simulink model "debugController"  (R2017a)
settings: Solver=VariableStepAuto  StartTime=0.0  StopTime=10.0  RelTol=1e-3
values from neighbouring files (symbols this model uses):
  k_bal = 10    [automatas_matlab.m]
  m_c = 50000    [automatas_matlab.m]
  m_l = 65000    [automatas_matlab.m]
  M_t = m_c + (J_w_t + J_m_t * r_t ^ 2)/ R_w_t ^ 2    (= 59008)    [automatas_matlab.m]
  n_bal = 3    [automatas_matlab.m]
undefined symbols (not defined in the file or in its folder): Ba_b, Ksa_b, lh
settings Model: Creator=laure  LastModifiedBy=laure

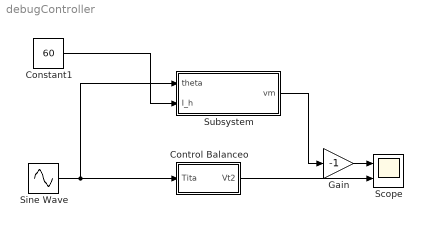
== system debugController ==
  Constant1 : Constant  Value=60
  Control Balanceo : Subsystem
  Gain : Gain  Gain=-1
  Scope : Scope  NumInputPorts=2
  Sine Wave : Sin  SampleTime=0
  Subsystem : Subsystem
  wires:
  Control Balanceo/1(Vt2) -> Scope/2
  Constant1/1 -> Subsystem/2(I_h)
  Sine Wave/1 -> Subsystem/1(theta), Control Balanceo/1(Tita)
  Subsystem/1(vm) -> Gain/1
  Gain/1 -> Scope/1

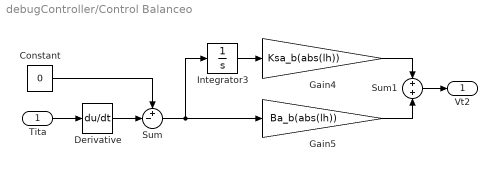
== system debugController/Control Balanceo ==
  Tita : Inport
  Constant : Constant  Value=0
  Derivative : Derivative
  Gain4 : Gain  Gain=Ksa_b(abs(lh))
  Gain5 : Gain  Gain=Ba_b(abs(lh))
  Integrator3 : Integrator
  Sum : Sum  Inputs=+-|
  Sum1 : Sum  Inputs=+|+
  Vt2 : Outport
  wires:
  Integrator3/1 -> Gain4/1
  Constant/1 -> Sum/1
  Tita/1 -> Derivative/1
  Derivative/1 -> Sum/2
  Gain4/1 -> Sum1/1
  Gain5/1 -> Sum1/2
  Sum1/1 -> Vt2/1
  Sum/1 -> Integrator3/1, Gain5/1

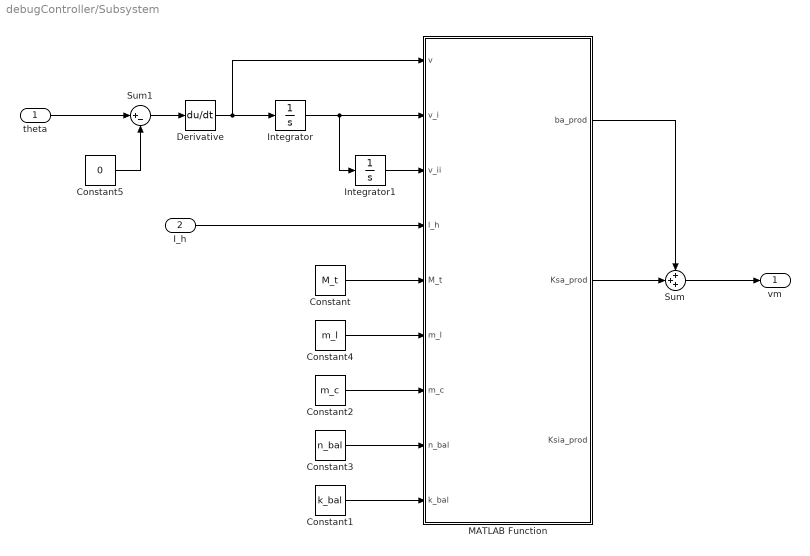
== system debugController/Subsystem ==
  theta : Inport
  I_h : Inport  Port=2
  Constant : Constant  Value=M_t
  Constant1 : Constant  Value=k_bal
  Constant2 : Constant  Value=m_c
  Constant3 : Constant  Value=n_bal
  Constant4 : Constant  Value=m_l
  Constant5 : Constant  Value=0
  Derivative : Derivative
  Integrator : Integrator
  Integrator1 : Integrator
  MATLAB Function : MATLAB Function  TreatAsAtomicUnit=on
  Sum : Sum  Inputs=+++
  Sum1 : Sum  Inputs=|+-
  vm : Outport
  wires:
  MATLAB Function/1(ba_prod) -> Sum/1
  I_h/1 -> MATLAB Function/4(l_h)
  MATLAB Function/2(Ksa_prod) -> Sum/2
  theta/1 -> Sum1/1
  Integrator/1 -> Integrator1/1, MATLAB Function/2(v_i)
  Sum/1 -> vm/1
  Integrator1/1 -> MATLAB Function/3(v_ii)
  Constant/1 -> MATLAB Function/5(M_t)
  Constant2/1 -> MATLAB Function/7(m_c)
  Constant3/1 -> MATLAB Function/8(n_bal)
  Constant1/1 -> MATLAB Function/9(k_bal)
  Constant4/1 -> MATLAB Function/6(m_l)
  Constant5/1 -> Sum1/2
  Sum1/1 -> Derivative/1
  Derivative/1 -> MATLAB Function/1(v), Integrator/1

== matlab function debugController/Subsystem/MATLAB Function ==
  data: ba_prod output; Ksa_prod output; Ksia_prod output; v input; v_i input; v_ii input; l_h input; M_t input; m_l input; m_c input; n_bal input; k_bal input
function [ba_prod, Ksa_prod, Ksia_prod] = fcn(v, v_i, v_ii, l_h, M_t, m_l, m_c, n_bal, k_bal)


poles = sqrt(complex(-M_t/ ((M_t + m_l)* l_h)))
w_n = abs(poles(1))

w_pos = k_bal * w_n

J_eq = - (M_t + m_l) * l_h /(m_c + m_l)

ba = J_eq * n_bal * w_pos
Ksa = J_eq * n_bal * w_pos ^ 2
Ksia = J_eq * w_pos ^ 3


ba_prod = ba * v
Ksa_prod = Ksa * v_i
Ksia_prod = Ksia * v_ii



end
